simulink model "MR6Simulinknodos"  (R2013a)
settings: Solver=VariableStepDiscrete  StartTime=0.0  StopTime=10.0  RelTol=1e-6
libraries: powerlib x37
settings Model: Creator=Erika  LastModifiedBy=Erika
settings SolverCC: AlgebraicLoopSolver=LineSearch

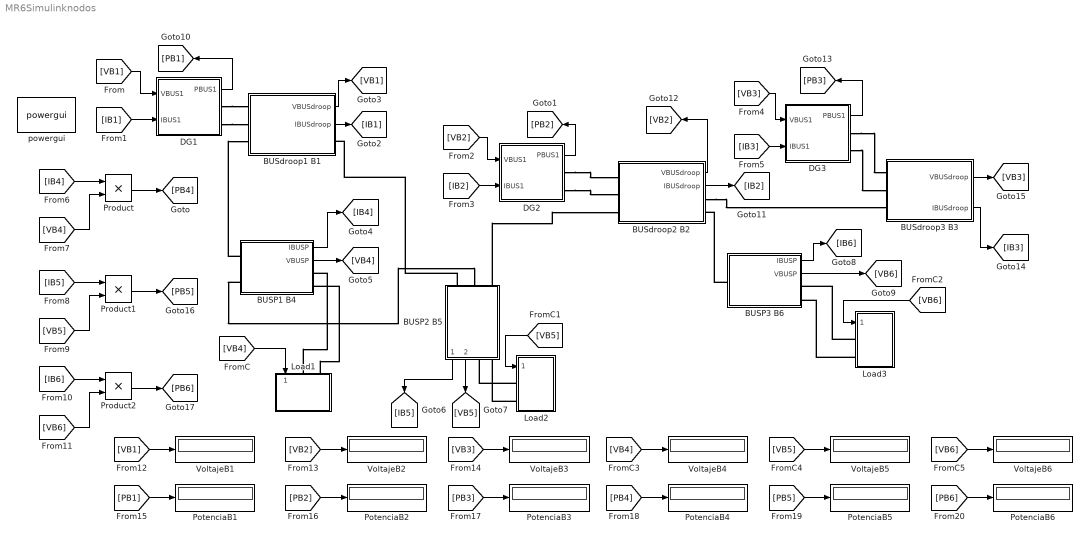
== system MR6Simulinknodos ==
  BUSP1 B4 : Subsystem
  BUSP2 B5 : Subsystem
  BUSP3 B6 : Subsystem
  BUSdroop1 B1 : Subsystem
  BUSdroop2 B2 : Subsystem
  BUSdroop3 B3 : Subsystem
  DG1 : Subsystem
  DG2 : Subsystem
  DG3 : Subsystem
  Load1 : Subsystem
  Load2 : Subsystem
  Load3 : Subsystem
  PotenciaB{1..5} (5 alike) : Display
  "PotenciaB6 " : Display
  Product : Product
  Product1 : Product
  Product2 : Product
  VoltajeB{1..2,4..6} (5 alike) : Display
  "VoltajeB3 " : Display
  powergui : powerlib/powergui  Priority=1  SimulationMode=Continuous  SolverType=Tustin  SampleTime=50e-6  frequency=60  SPID=off  DisableSnubberDevices=off  DisableRonSwitches=off  DisableVfSwitches=off  SwTol=0  Interpol=off  DisplayEquations=off  frequencyindice=0  Pbase=100e6  ErrMax=1e-4  Iterations=50  UnitsV=kV  UnitsW=MW  FunctionMessages=off  echomessages=off  HookPort=off  EnableUseOfTLC=off  x0status=blocks  RestoreLinks=warning  ResistiveCurrentMeasurement=off  Frange=[0:2:500]  Ylog=off  Xlog=on  ShowGrid=off  save=off  variable=ZData  ZoomFFT=off  StartTime=0.0  cycles=1  DisplayStyle=1  fundamental=60  FreqAxis=off  MaxFrequency=1000  frequencyindicesteady=1  RmsSteady=1  display=off  Ts=0  methode=off
  wires:
  [VB1] -> DG1/1(VBUS1)
  [IB1] -> DG1/2(IBUS1)
  DG1/1(PBUS1) -> [PB1]
  [VB4] -> Load1/1(VBUSc)
  BUSP1 B4/1(IBUSP) -> [IB4]
  BUSP1 B4/2(VBUSP) -> [VB4]
  [VB5] -> Load2/1(VBUSc)
  BUSP2 B5/1(IBUSP) -> [IB5]
  BUSP2 B5/2(VBUSP) -> [VB5]
  [VB6] -> Load3/1(VBUSc)
  BUSP3 B6/1(IBUSP) -> [IB6]
  BUSP3 B6/2(VBUSP) -> [VB6]
  BUSdroop1 B1/1(VBUSdroop) -> [VB1]
  BUSdroop1 B1/2(IBUSdroop) -> [IB1]
  [VB2] -> DG2/1(VBUS1)
  [IB2] -> DG2/2(IBUS1)
  DG2/1(PBUS1) -> [PB2]
  BUSdroop2 B2/1(VBUSdroop) -> [VB2]
  BUSdroop2 B2/2(IBUSdroop) -> [IB2]
  [VB3] -> DG3/1(VBUS1)
  [IB3] -> DG3/2(IBUS1)
  DG3/1(PBUS1) -> [PB3]
  BUSdroop3 B3/1(VBUSdroop) -> [VB3]
  BUSdroop3 B3/2(IBUSdroop) -> [IB3]
  [IB4] -> Product/1
  [VB4] -> Product/2
  Product/1 -> [PB4]
  [IB5] -> Product1/1
  [VB5] -> Product1/2
  Product1/1 -> [PB5]
  [IB6] -> Product2/1
  [VB6] -> Product2/2
  Product2/1 -> [PB6]
  [VB1] -> VoltajeB1/1
  [VB2] -> VoltajeB2/1
  [VB3] -> "VoltajeB3 "/1
  [VB4] -> VoltajeB4/1
  [VB5] -> VoltajeB5/1
  [VB6] -> VoltajeB6/1
  [PB1] -> PotenciaB1/1
  [PB2] -> PotenciaB2/1
  [PB3] -> PotenciaB3/1
  [PB4] -> PotenciaB4/1
  [PB5] -> PotenciaB5/1
  [PB6] -> "PotenciaB6 "/1
  connections:
  BUSP1 B4/LConn1 -- BUSdroop1 B1/LConn3
  BUSP1 B4/LConn2 -- BUSP2 B5/LConn2
  BUSP2 B5/LConn1 -- BUSdroop1 B1/RConn1
  BUSP2 B5/LConn3 -- BUSdroop2 B2/LConn3
  BUSdroop2 B2/RConn1 -- BUSdroop3 B3/LConn3
  BUSP3 B6/LConn1 -- BUSdroop2 B2/RConn2
  Load3/LConn1 -- BUSP3 B6/RConn1
  Load3/LConn2 -- BUSP3 B6/RConn2
  Load2/LConn1 -- BUSP2 B5/RConn1
  Load2/LConn2 -- BUSP2 B5/RConn2
  Load1/LConn1 -- BUSP1 B4/RConn1
  Load1/LConn2 -- BUSP1 B4/RConn2
  DG1/RConn1 -- BUSdroop1 B1/LConn1
  DG1/RConn2 -- BUSdroop1 B1/LConn2
  DG2/RConn1 -- BUSdroop2 B2/LConn1
  DG2/RConn2 -- BUSdroop2 B2/LConn2
  DG3/RConn2 -- BUSdroop3 B3/LConn2
  DG3/RConn1 -- BUSdroop3 B3/LConn1

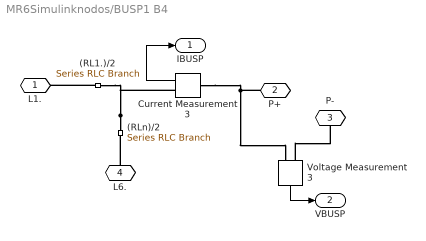
== system MR6Simulinknodos/BUSP1 B4 ==
  (RL1.)/2 : powerlib/Elements/Series RLC Branch  LConnTagsString=__new0  RConnTagsString=__new0  BranchType=R  Resistance=.041154  Inductance=1e-3  SetiL0=off  InitialCurrent=0  Capacitance=1e-6  Setx0=off  InitialVoltage=0  Measurements=None
  (RLn)/2 : powerlib/Elements/Series RLC Branch  LConnTagsString=__new0  RConnTagsString=__new0  BranchType=R  Resistance=.140068  Inductance=1e-3  SetiL0=off  InitialCurrent=0  Capacitance=1e-6  Setx0=off  InitialVoltage=0  Measurements=None
  Current Measurement3 : powerlib/Measurements/Current Measurement  PhasorSimulation=off  OutputType=Complex  PSBequivalent=0
  Voltage Measurement3 : powerlib/Measurements/Voltage Measurement  PhasorSimulation=off  OutputType=Complex  PSBequivalent=0
  L1. : PMIOPort  Port=1  Side=Left
  P+ : PMIOPort  Port=2  Side=Right
  P- : PMIOPort  Port=3  Side=Right
  L6. : PMIOPort  Port=4  Side=Left
  IBUSP : Outport
  VBUSP : Outport  Port=2
  wires:
  Current Measurement3/1 -> IBUSP/1
  Voltage Measurement3/1 -> VBUSP/1
  connections:
  Voltage Measurement3/LConn2 -- P-/RConn1
  L6./RConn1 -- (RLn)/2/RConn1
  (RL1.)/2/LConn1 -- L1./RConn1
  (RLn)/2/LConn1 -- Current Measurement3/RConn1 -- (RL1.)/2/RConn1
  Current Measurement3/LConn1 -- Voltage Measurement3/LConn1 -- P+/RConn1

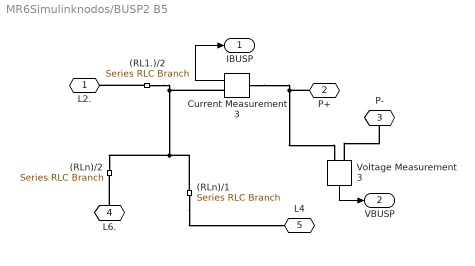
== system MR6Simulinknodos/BUSP2 B5 ==
  (RL1.)/2 : powerlib/Elements/Series RLC Branch  LConnTagsString=__new0  RConnTagsString=__new0  BranchType=R  Resistance=.096026  Inductance=1e-3  SetiL0=off  InitialCurrent=0  Capacitance=1e-6  Setx0=off  InitialVoltage=0  Measurements=None
  (RLn)/1 : powerlib/Elements/Series RLC Branch  LConnTagsString=__new0  RConnTagsString=__new0  BranchType=R  Resistance=.124906  Inductance=1e-3  SetiL0=off  InitialCurrent=0  Capacitance=1e-6  Setx0=off  InitialVoltage=0  Measurements=None
  (RLn)/2 : powerlib/Elements/Series RLC Branch  LConnTagsString=__new0  RConnTagsString=__new0  BranchType=R  Resistance=.140068  Inductance=1e-3  SetiL0=off  InitialCurrent=0  Capacitance=1e-6  Setx0=off  InitialVoltage=0  Measurements=None
  Current Measurement3 : powerlib/Measurements/Current Measurement  PhasorSimulation=off  OutputType=Complex  PSBequivalent=0
  Voltage Measurement3 : powerlib/Measurements/Voltage Measurement  PhasorSimulation=off  OutputType=Complex  PSBequivalent=0
  L2. : PMIOPort  Port=1  Side=Left
  P+ : PMIOPort  Port=2  Side=Right
  P- : PMIOPort  Port=3  Side=Right
  L6. : PMIOPort  Port=4  Side=Left
  L4 : PMIOPort  Port=5  Side=Left
  IBUSP : Outport
  VBUSP : Outport  Port=2
  wires:
  Voltage Measurement3/1 -> VBUSP/1
  Current Measurement3/1 -> IBUSP/1
  connections:
  P+/RConn1 -- Voltage Measurement3/LConn1 -- Current Measurement3/LConn1
  (RL1.)/2/RConn1 -- Current Measurement3/RConn1 -- (RLn)/2/LConn1 -- (RLn)/1/LConn1
  (RL1.)/2/LConn1 -- L2./RConn1
  L6./RConn1 -- (RLn)/2/RConn1
  Voltage Measurement3/LConn2 -- P-/RConn1
  (RLn)/1/RConn1 -- L4/RConn1

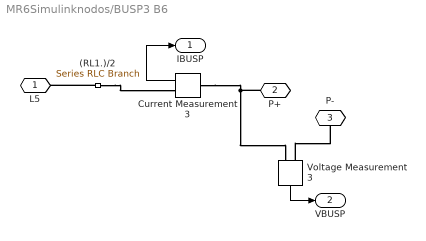
== system MR6Simulinknodos/BUSP3 B6 ==
  (RL1.)/2 : powerlib/Elements/Series RLC Branch  LConnTagsString=__new0  RConnTagsString=__new0  BranchType=R  Resistance=.2166  Inductance=1e-3  SetiL0=off  InitialCurrent=0  Capacitance=1e-6  Setx0=off  InitialVoltage=0  Measurements=None
  Current Measurement3 : powerlib/Measurements/Current Measurement  PhasorSimulation=off  OutputType=Complex  PSBequivalent=0
  Voltage Measurement3 : powerlib/Measurements/Voltage Measurement  PhasorSimulation=off  OutputType=Complex  PSBequivalent=0
  "L5 " : PMIOPort  Port=1  Side=Left
  P+ : PMIOPort  Port=2  Side=Right
  P- : PMIOPort  Port=3  Side=Right
  IBUSP : Outport
  VBUSP : Outport  Port=2
  wires:
  Current Measurement3/1 -> IBUSP/1
  Voltage Measurement3/1 -> VBUSP/1
  connections:
  Voltage Measurement3/LConn2 -- P-/RConn1
  (RL1.)/2/LConn1 -- "L5 "/RConn1
  (RL1.)/2/RConn1 -- Current Measurement3/RConn1
  Current Measurement3/LConn1 -- Voltage Measurement3/LConn1 -- P+/RConn1

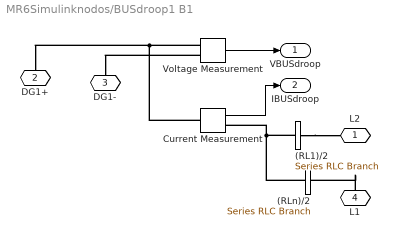
== system MR6Simulinknodos/BUSdroop1 B1 ==
  " (RL1)/2" : powerlib/Elements/Series RLC Branch  LConnTagsString=__new0  RConnTagsString=__new0  BranchType=R  Resistance=.096026  Inductance=1e-3  SetiL0=off  InitialCurrent=0  Capacitance=1e-6  Setx0=off  InitialVoltage=0  Measurements=None
  " (RLn)/2" : powerlib/Elements/Series RLC Branch  LConnTagsString=__new0  RConnTagsString=__new0  BranchType=R  Resistance=.041154  Inductance=1e-3  SetiL0=off  InitialCurrent=0  Capacitance=1e-6  Setx0=off  InitialVoltage=0  Measurements=None
  Current Measurement : powerlib/Measurements/Current Measurement  PhasorSimulation=off  OutputType=Complex  PSBequivalent=0
  Voltage Measurement : powerlib/Measurements/Voltage Measurement  PhasorSimulation=off  OutputType=Complex  PSBequivalent=0
  L2 : PMIOPort  Port=1  Side=Right
  DG1+ : PMIOPort  Port=2  Side=Left
  DG1- : PMIOPort  Port=3  Side=Left
  L1 : PMIOPort  Port=4  Side=Left
  VBUSdroop : Outport
  IBUSdroop : Outport  Port=2
  wires:
  Current Measurement/1 -> IBUSdroop/1
  Voltage Measurement/1 -> VBUSdroop/1
  connections:
  Voltage Measurement/LConn2 -- DG1-/RConn1
  L1/RConn1 -- " (RLn)/2"/RConn1
  " (RL1)/2"/LConn1 -- Current Measurement/RConn1 -- " (RLn)/2"/LConn1
  Voltage Measurement/LConn1 -- DG1+/RConn1 -- Current Measurement/LConn1
  " (RL1)/2"/RConn1 -- L2/RConn1

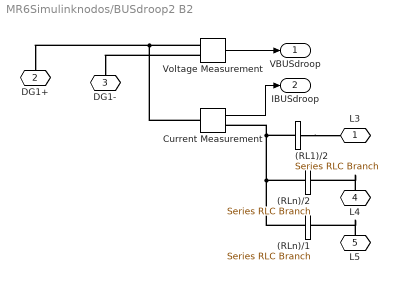
== system MR6Simulinknodos/BUSdroop2 B2 ==
  " (RL1)/2" : powerlib/Elements/Series RLC Branch  LConnTagsString=__new0  RConnTagsString=__new0  BranchType=R  Resistance=.23103  Inductance=1e-3  SetiL0=off  InitialCurrent=0  Capacitance=1e-6  Setx0=off  InitialVoltage=0  Measurements=None
  " (RLn)/1" : powerlib/Elements/Series RLC Branch  LConnTagsString=__new0  RConnTagsString=__new0  BranchType=R  Resistance=.2166  Inductance=1e-3  SetiL0=off  InitialCurrent=0  Capacitance=1e-6  Setx0=off  InitialVoltage=0  Measurements=None
  " (RLn)/2" : powerlib/Elements/Series RLC Branch  LConnTagsString=__new0  RConnTagsString=__new0  BranchType=R  Resistance=.124906  Inductance=1e-3  SetiL0=off  InitialCurrent=0  Capacitance=1e-6  Setx0=off  InitialVoltage=0  Measurements=None
  Current Measurement : powerlib/Measurements/Current Measurement  PhasorSimulation=off  OutputType=Complex  PSBequivalent=0
  Voltage Measurement : powerlib/Measurements/Voltage Measurement  PhasorSimulation=off  OutputType=Complex  PSBequivalent=0
  L3 : PMIOPort  Port=1  Side=Right
  DG1+ : PMIOPort  Port=2  Side=Left
  DG1- : PMIOPort  Port=3  Side=Left
  L4 : PMIOPort  Port=4  Side=Left
  L5 : PMIOPort  Port=5  Side=Right
  VBUSdroop : Outport
  IBUSdroop : Outport  Port=2
  wires:
  Voltage Measurement/1 -> VBUSdroop/1
  Current Measurement/1 -> IBUSdroop/1
  connections:
  " (RL1)/2"/RConn1 -- L3/RConn1
  Current Measurement/LConn1 -- DG1+/RConn1 -- Voltage Measurement/LConn1
  " (RLn)/2"/LConn1 -- Current Measurement/RConn1 -- " (RL1)/2"/LConn1 -- " (RLn)/1"/LConn1
  L4/RConn1 -- " (RLn)/2"/RConn1
  Voltage Measurement/LConn2 -- DG1-/RConn1
  L5/RConn1 -- " (RLn)/1"/RConn1

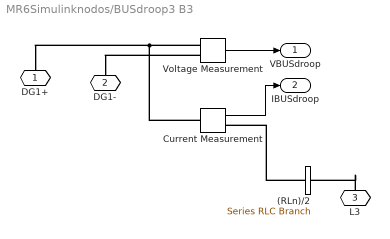
== system MR6Simulinknodos/BUSdroop3 B3 ==
  " (RLn)/2" : powerlib/Elements/Series RLC Branch  LConnTagsString=__new0  RConnTagsString=__new0  BranchType=R  Resistance=.23103  Inductance=1e-3  SetiL0=off  InitialCurrent=0  Capacitance=1e-6  Setx0=off  InitialVoltage=0  Measurements=None
  Current Measurement : powerlib/Measurements/Current Measurement  PhasorSimulation=off  OutputType=Complex  PSBequivalent=0
  Voltage Measurement : powerlib/Measurements/Voltage Measurement  PhasorSimulation=off  OutputType=Complex  PSBequivalent=0
  DG1+ : PMIOPort  Port=1  Side=Left
  DG1- : PMIOPort  Port=2  Side=Left
  L3 : PMIOPort  Port=3  Side=Left
  VBUSdroop : Outport
  IBUSdroop : Outport  Port=2
  wires:
  Current Measurement/1 -> IBUSdroop/1
  Voltage Measurement/1 -> VBUSdroop/1
  connections:
  Voltage Measurement/LConn2 -- DG1-/RConn1
  L3/RConn1 -- " (RLn)/2"/RConn1
  " (RLn)/2"/LConn1 -- Current Measurement/RConn1
  Voltage Measurement/LConn1 -- DG1+/RConn1 -- Current Measurement/LConn1

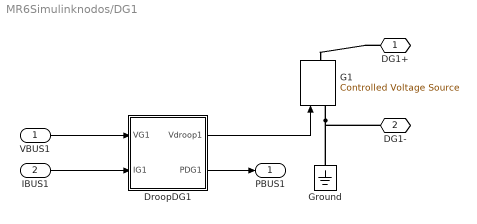
== system MR6Simulinknodos/DG1 ==
  VBUS1 : Inport
  IBUS1 : Inport  Port=2
  DroopDG1 : Subsystem
  G1 : powerlib/Electrical Sources/Controlled Voltage Source  Initialize=on  Source_Type=DC  Amplitude=380  Phase=0  Frequency=0  Measurements=None
  Ground : powerlib/Elements/Ground  LConnTagsString=a
  DG1+ : PMIOPort  Port=1  Side=Right
  DG1- : PMIOPort  Port=2  Side=Right
  PBUS1 : Outport
  wires:
  DroopDG1/1(Vdroop1) -> G1/1
  DroopDG1/2(PDG1) -> PBUS1/1
  IBUS1/1 -> DroopDG1/2(IG1)
  VBUS1/1 -> DroopDG1/1(VG1)
  connections:
  G1/LConn1 -- DG1-/RConn1 -- Ground/LConn1
  DG1+/RConn1 -- G1/RConn1

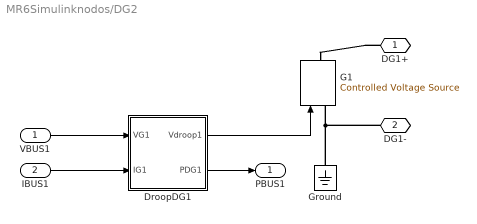
== system MR6Simulinknodos/DG2 ==
  VBUS1 : Inport
  IBUS1 : Inport  Port=2
  DroopDG1 : Subsystem
  G1 : powerlib/Electrical Sources/Controlled Voltage Source  Initialize=on  Source_Type=DC  Amplitude=380  Phase=0  Frequency=0  Measurements=None
  Ground : powerlib/Elements/Ground  LConnTagsString=a
  DG1+ : PMIOPort  Port=1  Side=Right
  DG1- : PMIOPort  Port=2  Side=Right
  PBUS1 : Outport
  wires:
  VBUS1/1 -> DroopDG1/1(VG1)
  IBUS1/1 -> DroopDG1/2(IG1)
  DroopDG1/2(PDG1) -> PBUS1/1
  DroopDG1/1(Vdroop1) -> G1/1
  connections:
  DG1+/RConn1 -- G1/RConn1
  Ground/LConn1 -- DG1-/RConn1 -- G1/LConn1

== system MR6Simulinknodos/DG3 ==
  VBUS1 : Inport
  IBUS1 : Inport  Port=2
  DroopDG1 : Subsystem
  G1 : powerlib/Electrical Sources/Controlled Voltage Source  Initialize=on  Source_Type=DC  Amplitude=380  Phase=0  Frequency=0  Measurements=None
  Ground : powerlib/Elements/Ground  LConnTagsString=a
  DG1+ : PMIOPort  Port=1  Side=Right
  DG1- : PMIOPort  Port=2  Side=Right
  PBUS1 : Outport
  wires:
  DroopDG1/1(Vdroop1) -> G1/1
  DroopDG1/2(PDG1) -> PBUS1/1
  IBUS1/1 -> DroopDG1/2(IG1)
  VBUS1/1 -> DroopDG1/1(VG1)
  connections:
  G1/LConn1 -- DG1-/RConn1 -- Ground/LConn1
  DG1+/RConn1 -- G1/RConn1

== system MR6Simulinknodos/Load1 ==
  VBUSc : Inport
  Constant4 : Constant  Value=14000
  Controlled Current Source : powerlib/Electrical Sources/Controlled Current Source  Initialize=off  Source_Type=DC  Amplitude=0  Phase=0  Frequency=0  Measurements=None
  Divide2 : Product  Inputs=*/
  Ground3 : powerlib/Elements/Ground  LConnTagsString=a
  Load1+ : PMIOPort  Port=1  Side=Left
  Load1- : PMIOPort  Port=2  Side=Left
  wires:
  Constant4/1 -> Divide2/1
  Divide2/1 -> Controlled Current Source/1
  VBUSc/1 -> Divide2/2
  connections:
  Controlled Current Source/RConn1 -- Load1-/RConn1 -- Ground3/LConn1
  Controlled Current Source/LConn1 -- Load1+/RConn1

== system MR6Simulinknodos/Load2 ==
  VBUSc : Inport
  Constant4 : Constant  Value=8000
  Controlled Current Source : powerlib/Electrical Sources/Controlled Current Source  Initialize=off  Source_Type=DC  Amplitude=0  Phase=0  Frequency=0  Measurements=None
  Divide2 : Product  Inputs=*/
  Ground3 : powerlib/Elements/Ground  LConnTagsString=a
  Load1+ : PMIOPort  Port=1  Side=Left
  Load1- : PMIOPort  Port=2  Side=Left
  wires:
  VBUSc/1 -> Divide2/2
  Divide2/1 -> Controlled Current Source/1
  Constant4/1 -> Divide2/1
  connections:
  Controlled Current Source/LConn1 -- Load1+/RConn1
  Ground3/LConn1 -- Load1-/RConn1 -- Controlled Current Source/RConn1

== system MR6Simulinknodos/Load3 ==
  VBUSc : Inport
  Constant4 : Constant  Value=7000
  Controlled Current Source : powerlib/Electrical Sources/Controlled Current Source  Initialize=off  Source_Type=DC  Amplitude=0  Phase=0  Frequency=0  Measurements=None
  Divide2 : Product  Inputs=*/
  Ground3 : powerlib/Elements/Ground  LConnTagsString=a
  Load1+ : PMIOPort  Port=1  Side=Left
  Load1- : PMIOPort  Port=2  Side=Left
  wires:
  Constant4/1 -> Divide2/1
  Divide2/1 -> Controlled Current Source/1
  VBUSc/1 -> Divide2/2
  connections:
  Controlled Current Source/RConn1 -- Load1-/RConn1 -- Ground3/LConn1
  Controlled Current Source/LConn1 -- Load1+/RConn1

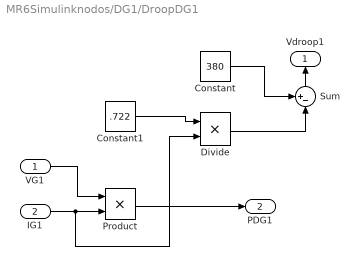
== system MR6Simulinknodos/DG1/DroopDG1 ==
  VG1 : Inport
  IG1 : Inport  Port=2
  Constant : Constant  Value=380
  Constant1 : Constant  Value=.722
  Divide : Product  Inputs=**
  Product : Product
  Sum : Sum  Inputs=+-|
  Vdroop1 : Outport
  PDG1 : Outport  Port=2
  wires:
  Constant1/1 -> Divide/1
  IG1/1 -> Divide/2, Product/2
  Constant/1 -> Sum/1
  Sum/1 -> Vdroop1/1
  Divide/1 -> Sum/2
  Product/1 -> PDG1/1
  VG1/1 -> Product/1

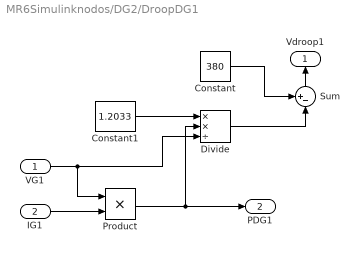
== system MR6Simulinknodos/DG2/DroopDG1 ==
  VG1 : Inport
  IG1 : Inport  Port=2
  Constant : Constant  Value=380
  Constant1 : Constant  Value=1.2033
  Divide : Product  Inputs=**/
  Product : Product
  Sum : Sum  Inputs=+-|
  Vdroop1 : Outport
  PDG1 : Outport  Port=2
  wires:
  Product/1 -> PDG1/1, Divide/2
  VG1/1 -> Divide/3, Product/1
  Divide/1 -> Sum/2
  Sum/1 -> Vdroop1/1
  Constant/1 -> Sum/1
  IG1/1 -> Product/2
  Constant1/1 -> Divide/1

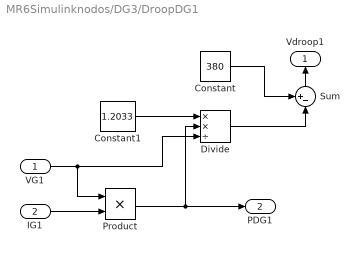
== system MR6Simulinknodos/DG3/DroopDG1 ==
  VG1 : Inport
  IG1 : Inport  Port=2
  Constant : Constant  Value=380
  Constant1 : Constant  Value=1.2033
  Divide : Product  Inputs=**/
  Product : Product
  Sum : Sum  Inputs=+-|
  Vdroop1 : Outport
  PDG1 : Outport  Port=2
  wires:
  Constant1/1 -> Divide/1
  IG1/1 -> Product/2
  Constant/1 -> Sum/1
  Sum/1 -> Vdroop1/1
  Divide/1 -> Sum/2
  VG1/1 -> Product/1, Divide/3
  Product/1 -> Divide/2, PDG1/1
